simulink model "dynamics_reduced"  (Simulink 7.4)
settings: Solver=ode45  StartTime=0.0  StopTime=10.0  RelTol=1e-3
undefined symbols (not defined in the file or in its folder): boom, f1, f2, f3, f4, f5, I_x, I_y, I_z, phi0, r_phi0, r_psi0, r_theta0, theta0
libraries: Copter_Library x5
settings Model: Creator=Alex  LastModifiedBy=Alex

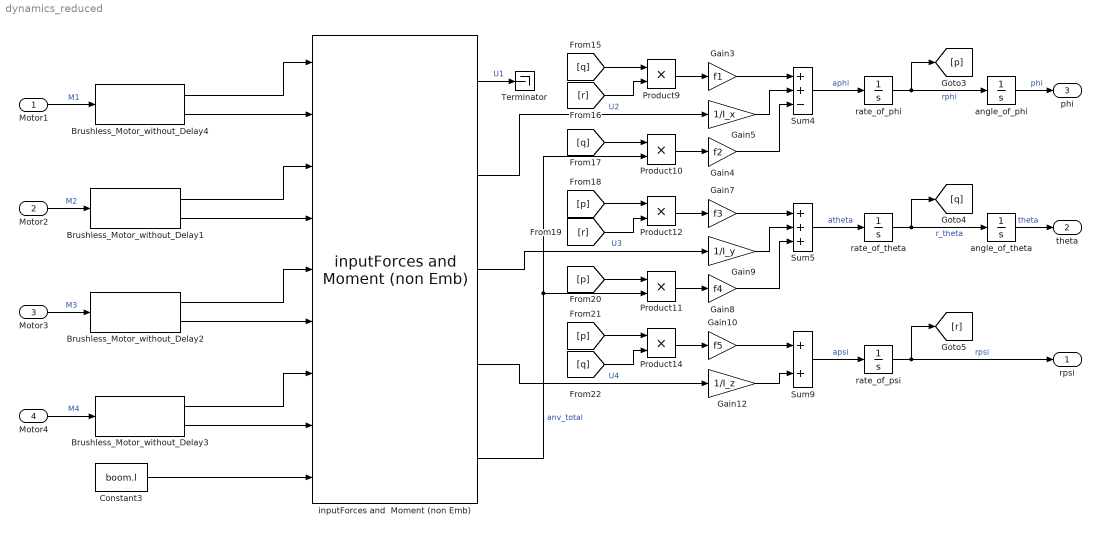
== system dynamics_reduced ==
  Motor1 : Inport  OutDataType=fixdt(1, 16)  OutScaling=2^0
  Motor2 : Inport  Port=2  OutDataType=fixdt(1, 16)  OutScaling=2^0
  Motor3 : Inport  Port=3  OutDataType=fixdt(1, 16)  OutScaling=2^0
  Motor4 : Inport  Port=4  OutDataType=fixdt(1, 16)  OutScaling=2^0
  Brushless_Motor_without_Delay{1..4} (4 alike) : Copter_Library/Brushless_Motor_without_Delay  SystemSampleTime=-1  M_error=0.99
  Constant3 : Constant  Value=boom.l
  Gain10 : Gain  Gain=f5
  Gain12 : Gain  Gain=1/I_z
  Gain3 : Gain  Gain=f1
  Gain4 : Gain  Gain=f2
  Gain5 : Gain  Gain=1/I_x
  Gain7 : Gain  Gain=f3
  Gain8 : Gain  Gain=f4
  Gain9 : Gain  Gain=1/I_y
  Product{9..12,14} (5 alike) : Product  RndMeth=Zero
  Sum4 : Sum  Inputs=++-
  Sum5 : Sum  Inputs=+++
  Sum9 : Sum
  Terminator : Terminator
  angle_of_phi : Integrator  InitialCondition=phi0
  angle_of_theta : Integrator  InitialCondition=theta0
  inputForces and  Moment (non Emb) : Copter_Library/inputForces and  Moment (non Emb)  SystemSampleTime=-1
  rate_of_phi : Integrator  InitialCondition=r_phi0
  rate_of_psi : Integrator  InitialCondition=r_psi0
  rate_of_theta : Integrator  InitialCondition=r_theta0
  rpsi : Outport
  theta : Outport  Port=2
  phi : Outport  Port=3
  wires:
  Motor4/1 -> Brushless_Motor_without_Delay3/1  "M4"
  Motor2/1 -> Brushless_Motor_without_Delay1/1  "M2"
  Motor1/1 -> Brushless_Motor_without_Delay4/1  "M1"
  Motor3/1 -> Brushless_Motor_without_Delay2/1  "M3"
  Constant3/1 -> inputForces and  Moment (non Emb)/9
  inputForces and  Moment (non Emb)/4 -> Gain12/1  "U4"
  Product14/1 -> Gain10/1
  [q] -> Product14/2
  [p] -> Product14/1
  inputForces and  Moment (non Emb)/3 -> Gain9/1  "U3"
  Product11/1 -> Gain8/1
  [p] -> Product11/1
  Product12/1 -> Gain7/1
  [r] -> Product12/2
  [p] -> Product12/1
  inputForces and  Moment (non Emb)/2 -> Gain5/1  "U2"
  Product10/1 -> Gain4/1
  [q] -> Product10/1
  Product9/1 -> Gain3/1
  [r] -> Product9/2
  [q] -> Product9/1
  inputForces and  Moment (non Emb)/5 -> Product11/2, Product10/2  "anv_total"
  Brushless_Motor_without_Delay4/1 -> inputForces and  Moment (non Emb)/1
  Brushless_Motor_without_Delay1/1 -> inputForces and  Moment (non Emb)/3
  Brushless_Motor_without_Delay1/2 -> inputForces and  Moment (non Emb)/4
  Brushless_Motor_without_Delay2/1 -> inputForces and  Moment (non Emb)/5
  Brushless_Motor_without_Delay2/2 -> inputForces and  Moment (non Emb)/6
  Brushless_Motor_without_Delay3/1 -> inputForces and  Moment (non Emb)/7
  Brushless_Motor_without_Delay3/2 -> inputForces and  Moment (non Emb)/8
  Sum9/1 -> rate_of_psi/1  "apsi"
  Gain12/1 -> Sum9/2
  Gain10/1 -> Sum9/1
  Sum5/1 -> rate_of_theta/1  "atheta"
  Gain9/1 -> Sum5/2
  Gain7/1 -> Sum5/1
  Sum4/1 -> rate_of_phi/1  "aphi"
  Gain5/1 -> Sum4/2
  Gain3/1 -> Sum4/1
  angle_of_phi/1 -> phi/1  "phi"
  angle_of_theta/1 -> theta/1  "theta"
  rate_of_phi/1 -> [p], angle_of_phi/1  "rphi"
  rate_of_theta/1 -> angle_of_theta/1, [q]  "r_theta"
  rate_of_psi/1 -> [r], rpsi/1  "rpsi"
  Gain4/1 -> Sum4/3
  Gain8/1 -> Sum5/3
  inputForces and  Moment (non Emb)/1 -> Terminator/1  "U1"
  Brushless_Motor_without_Delay4/2 -> inputForces and  Moment (non Emb)/2
